simulink model "Non_Passivity"  (R2019b)
settings: Solver=FixedStepAuto  StartTime=0.0  StopTime=10  FixedStep=0.01  RelTol=1e-3
settings Model: Creator=김태욱  LastModifiedBy=김태욱

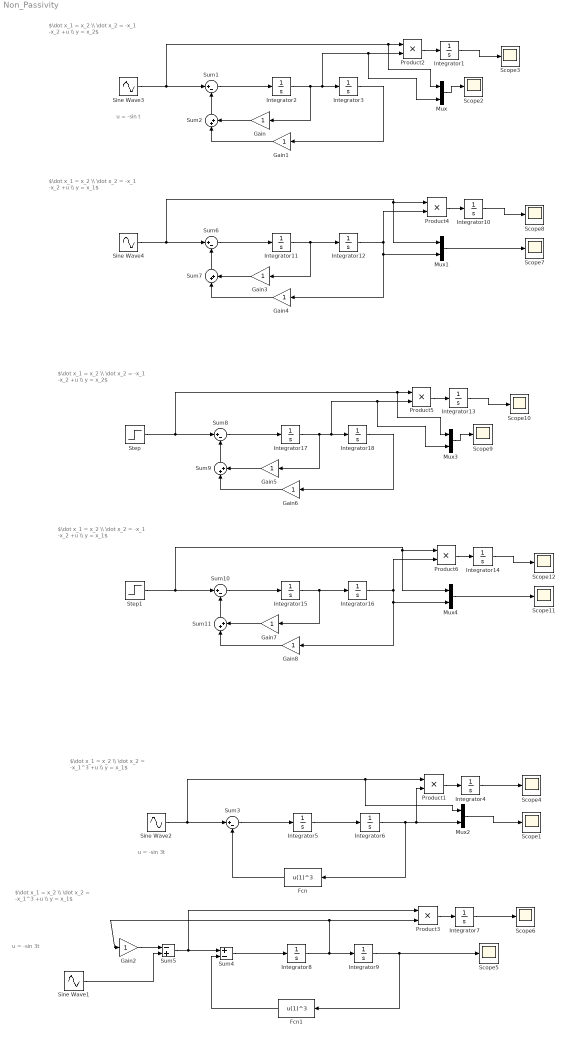
== system Non_Passivity ==
  note: u = -sin t
  note: $\dot x_1 = x_2 \\ \dot x_2 = -x_1 -x_2 +u \\ y = x_2$
  note: u = -sin 3t
  note: $\dot x_1 = x_2 \\ \dot x_2 = -x_1^3 +u \\ y = x_1$
  note: u = -sin 3t
  note: $\dot x_1 = x_2 \\ \dot x_2 = -x_1^3 +u \\ y = x_1$
  note: $\dot x_1 = x_2 \\ \dot x_2 = -x_1 -x_2 +u \\ y = x_1$
  note: $\dot x_1 = x_2 \\ \dot x_2 = -x_1 -x_2 +u \\ y = x_2$
  note: $\dot x_1 = x_2 \\ \dot x_2 = -x_1 -x_2 +u \\ y = x_1$
  Fcn : Fcn  Expr=u(1)^3
  Fcn1 : Fcn  Expr=u(1)^3
  Gain{,1..8} (9 alike) : Gain
  Integrator{1..4,7..18} (16 alike) : Integrator
  Integrator5 : Integrator  ContinuousStateAttributes='x1'
  Integrator6 : Integrator  ContinuousStateAttributes='x1'
  Mux{,1..4} (5 alike) : Mux  Inputs=2
  Product{1..6} (6 alike) : Product
  Scope{1..12} (12 alike) : Scope
  Sine Wave1 : Sin  Frequency=3  SampleTime=0
  Sine Wave2 : Sin  Amplitude=-1  SampleTime=0
  Sine Wave3 : Sin  Amplitude=-1  SampleTime=0
  Sine Wave4 : Sin  Amplitude=-1  Frequency=3  SampleTime=0
  Step : Step  SampleTime=0
  Step1 : Step  SampleTime=0
  Sum{1,3,6,8,10} (5 alike) : Sum  Inputs=|+-
  Sum{2,7,9,11} (4 alike) : Sum  Inputs=|++
  Sum4 : Sum  Inputs=+-
  Sum5 : Sum  Inputs=-+
  wires:
  Integrator2/1 -> Gain/1, Mux/2, Product2/2, Integrator3/1
  Sum1/1 -> Integrator2/1
  Integrator3/1 -> Gain1/1
  Product2/1 -> Integrator1/1
  Integrator1/1 -> Scope3/1
  Sine Wave3/1 -> Mux/1, Product2/1, Sum1/1
  Gain1/1 -> Sum2/1
  Sum2/1 -> Sum1/2
  Gain/1 -> Sum2/2
  Sine Wave2/1 -> Sum3/1, Mux2/1, Product1/1
  Integrator4/1 -> Scope4/1
  Product1/1 -> Integrator4/1
  Integrator6/1 -> Mux2/2, Product1/2, Fcn/1
  Sum3/1 -> Integrator5/1
  Integrator5/1 -> Integrator6/1
  Fcn/1 -> Sum3/2
  Sum4/1 -> Integrator8/1
  Integrator9/1 -> Scope5/1, Fcn1/1
  Product3/1 -> Integrator7/1
  Integrator7/1 -> Scope6/1
  Fcn1/1 -> Sum4/2
  Sine Wave1/1 -> Sum5/2
  Sum5/1 -> Product3/1, Sum4/1
  Gain2/1 -> Sum5/1
  Integrator8/1 -> Gain2/1, Product3/2, Integrator9/1
  Mux/1 -> Scope2/1
  Mux1/1 -> Scope7/1
  Gain3/1 -> Sum7/2
  Sum7/1 -> Sum6/2
  Gain4/1 -> Sum7/1
  Sine Wave4/1 -> Sum6/1, Mux1/1, Product4/1
  Integrator10/1 -> Scope8/1
  Product4/1 -> Integrator10/1
  Integrator12/1 -> Product4/2, Mux1/2, Gain4/1
  Sum6/1 -> Integrator11/1
  Integrator11/1 -> Integrator12/1, Gain3/1
  Mux2/1 -> Scope1/1
  Integrator15/1 -> Gain7/1, Integrator16/1
  Sum10/1 -> Integrator15/1
  Integrator16/1 -> Gain8/1, Mux4/2, Product6/2
  Product6/1 -> Integrator14/1
  Integrator14/1 -> Scope12/1
  Step1/1 -> Product6/1, Mux4/1, Sum10/1
  Gain8/1 -> Sum11/1
  Sum11/1 -> Sum10/2
  Gain7/1 -> Sum11/2
  Mux4/1 -> Scope11/1
  Mux3/1 -> Scope9/1
  Gain5/1 -> Sum9/2
  Sum9/1 -> Sum8/2
  Gain6/1 -> Sum9/1
  Step/1 -> Sum8/1, Product5/1, Mux3/1
  Integrator13/1 -> Scope10/1
  Product5/1 -> Integrator13/1
  Integrator18/1 -> Gain6/1
  Sum8/1 -> Integrator17/1
  Integrator17/1 -> Integrator18/1, Product5/2, Mux3/2, Gain5/1
